simulink model "test_mdl1"  (R2023a)
settings: Solver=VariableStepAuto  StartTime=0.0  StopTime=10.0  RelTol=1e-3
(part 2 of 8)

== system test_mdl1/VehicleCAN/ABS_ESC/ABS_Rapid_Data_Response_2 ==
  UUDTABSResponse2 : Constant  Value=0
  bus_creator : BusCreator  Inputs=1
  out_port : Outport
  wires:
  bus_creator/1 -> out_port/1  "test_mdl1"
  UUDTABSResponse2/1 -> bus_creator/1  "UUDTABSResponse2"

== system test_mdl1/VehicleCAN/ABS_ESC/ActiveFronSteering_Req ==
  SteWhlBrkAnRq_No_Cnt : Constant  Value=0
  SteWhlBrkAnRq_No_Cs : Constant  Value=0
  SteWhlBrkOffst_An_Rq : Constant  Value=0
  bus_creator : BusCreator  Inputs=3
  out_port : Outport
  wires:
  bus_creator/1 -> out_port/1  "test_mdl1"
  SteWhlBrkAnRq_No_Cnt/1 -> bus_creator/1  "SteWhlBrkAnRq_No_Cnt"
  SteWhlBrkAnRq_No_Cs/1 -> bus_creator/2  "SteWhlBrkAnRq_No_Cs"
  SteWhlBrkOffst_An_Rq/1 -> bus_creator/3  "SteWhlBrkOffst_An_Rq"

== system test_mdl1/VehicleCAN/ABS_ESC/BrakeSnData_3 ==
  VehLatComp_A_Actl : Constant  Value=0
  VehLongComp_A_Actl : Constant  Value=0
  VehOverGnd_V_Est : Constant  Value=0
  VehTrvlDir_D_Stat : Constant  Value=0
  VehYawComp_W_Actl : Constant  Value=0
  bus_creator : BusCreator  Inputs=5
  out_port : Outport
  wires:
  bus_creator/1 -> out_port/1  "test_mdl1"
  VehLatComp_A_Actl/1 -> bus_creator/1  "VehLatComp_A_Actl"
  VehLongComp_A_Actl/1 -> bus_creator/2  "VehLongComp_A_Actl"
  VehOverGnd_V_Est/1 -> bus_creator/3  "VehOverGnd_V_Est"
  VehTrvlDir_D_Stat/1 -> bus_creator/4  "VehTrvlDir_D_Stat"
  VehYawComp_W_Actl/1 -> bus_creator/5  "VehYawComp_W_Actl"

== system test_mdl1/VehicleCAN/ABS_ESC/BrakeSnData_4 ==
  BrkTotTqRqArb_No_Cnt : Constant  Value=0
  BrkTotTqRqArb_No_Cs : Constant  Value=0
  BrkTot_Tq_Actl : Constant  Value=0
  BrkTot_Tq_RqArb : Constant  Value=0
  HsaStat_D_Actl : Constant  Value=0
  VehRolComp_W_Actl : Constant  Value=0
  VehVertComp_A_Actl : Constant  Value=0
  bus_creator : BusCreator  Inputs=7
  out_port : Outport
  wires:
  bus_creator/1 -> out_port/1  "test_mdl1"
  BrkTotTqRqArb_No_Cnt/1 -> bus_creator/1  "BrkTotTqRqArb_No_Cnt"
  BrkTotTqRqArb_No_Cs/1 -> bus_creator/2  "BrkTotTqRqArb_No_Cs"
  BrkTot_Tq_Actl/1 -> bus_creator/3  "BrkTot_Tq_Actl"
  BrkTot_Tq_RqArb/1 -> bus_creator/4  "BrkTot_Tq_RqArb"
  HsaStat_D_Actl/1 -> bus_creator/5  "HsaStat_D_Actl"
  VehRolComp_W_Actl/1 -> bus_creator/6  "VehRolComp_W_Actl"
  VehVertComp_A_Actl/1 -> bus_creator/7  "VehVertComp_A_Actl"

== system test_mdl1/VehicleCAN/ABS_ESC/BrakeSnData_5 ==
  AwdLck_Tq_RqMn : Constant  Value=0
  AwdLck_Tq_RqMx : Constant  Value=0
  BrkCtrFnd_B_Stat : Constant  Value=0
  DrvSte_D_Stat : Constant  Value=0
  DrvSte_Tq_Rq : Constant  Value=0
  EmgcyBrkLamp_D_Rq : Constant  Value=0
  StopLamp_B_RqBrk : Constant  Value=0
  bus_creator : BusCreator  Inputs=7
  out_port : Outport
  wires:
  bus_creator/1 -> out_port/1  "test_mdl1"
  AwdLck_Tq_RqMn/1 -> bus_creator/1  "AwdLck_Tq_RqMn"
  AwdLck_Tq_RqMx/1 -> bus_creator/2  "AwdLck_Tq_RqMx"
  BrkCtrFnd_B_Stat/1 -> bus_creator/3  "BrkCtrFnd_B_Stat"
  DrvSte_D_Stat/1 -> bus_creator/4  "DrvSte_D_Stat"
  DrvSte_Tq_Rq/1 -> bus_creator/5  "DrvSte_Tq_Rq"
  EmgcyBrkLamp_D_Rq/1 -> bus_creator/6  "EmgcyBrkLamp_D_Rq"
  StopLamp_B_RqBrk/1 -> bus_creator/7  "StopLamp_B_RqBrk"

== system test_mdl1/VehicleCAN/ABS_ESC/BrakeSnData_6 ==
  StePinOffst_An_Est : Constant  Value=0
  StePinOffst_D_Stat : Constant  Value=0
  StePinOffst_No_Cnt : Constant  Value=0
  StePinOffst_No_Cs : Constant  Value=0
  bus_creator : BusCreator  Inputs=4
  out_port : Outport
  wires:
  bus_creator/1 -> out_port/1  "test_mdl1"
  StePinOffst_An_Est/1 -> bus_creator/1  "StePinOffst_An_Est"
  StePinOffst_D_Stat/1 -> bus_creator/2  "StePinOffst_D_Stat"
  StePinOffst_No_Cnt/1 -> bus_creator/3  "StePinOffst_No_Cnt"
  StePinOffst_No_Cs/1 -> bus_creator/4  "StePinOffst_No_Cs"

== system test_mdl1/VehicleCAN/ABS_ESC/BrakeSysFeatures ==
  BrkFluidLvl_D_Stat : Constant  Value=0
  LsmcBrkDecel_D_Stat : Constant  Value=0
  VehStab_D_Stat : Constant  Value=0
  VehVActlBrk_D_Qf : Constant  Value=0
  VehVActlBrk_No_Cnt : Constant  Value=0
  VehVActlBrk_No_Cs : Constant  Value=0
  VehYawLin_W_Rq : Constant  Value=0
  VehYawNonLin_W_Rq : Constant  Value=0
  Veh_V_ActlBrk : Constant  Value=0
  bus_creator : BusCreator  Inputs=9
  out_port : Outport
  wires:
  bus_creator/1 -> out_port/1  "test_mdl1"
  BrkFluidLvl_D_Stat/1 -> bus_creator/1  "BrkFluidLvl_D_Stat"
  LsmcBrkDecel_D_Stat/1 -> bus_creator/2  "LsmcBrkDecel_D_Stat"
  VehStab_D_Stat/1 -> bus_creator/3  "VehStab_D_Stat"
  VehVActlBrk_D_Qf/1 -> bus_creator/4  "VehVActlBrk_D_Qf"
  VehVActlBrk_No_Cnt/1 -> bus_creator/5  "VehVActlBrk_No_Cnt"
  VehVActlBrk_No_Cs/1 -> bus_creator/6  "VehVActlBrk_No_Cs"
  VehYawLin_W_Rq/1 -> bus_creator/7  "VehYawLin_W_Rq"
  VehYawNonLin_W_Rq/1 -> bus_creator/8  "VehYawNonLin_W_Rq"
  Veh_V_ActlBrk/1 -> bus_creator/9  "Veh_V_ActlBrk"

== system test_mdl1/VehicleCAN/ABS_ESC/BrakeSysFeatures_2 ==
  Abs_B_Falt : Constant  Value=0
  BpedMove_D_Actl : Constant  Value=0
  BpedMove_No_Cnt : Constant  Value=0
  BrkBstrVac_B_Rq : Constant  Value=0
  BrkLamp_B_Rq : Constant  Value=0
  ChimeBrk_B_Rq : Constant  Value=0
  DrvAntiLckLamp_D_Rq : Constant  Value=0
  DrvHdcLampInfo_D_Rq : Constant  Value=0
  DrvHdcMsg_D_Rq : Constant  Value=0
  DrvHdcWarnInfo_D_Rq : Constant  Value=0
  DrvSlipCtlLamp_D_Rq : Constant  Value=0
  DrvSlipCtlMde_D_Ind : Constant  Value=0
  HILL_DESC_MC : Constant  Value=0
  HdcMde_D_Actl : Constant  Value=0
  HsaMde_D_Mem : Constant  Value=0
  RearDiffElckrOpen_B_Rq : Constant  Value=0
  RearDiffLck_Tq2_RqMx : Constant  Value=0
  StabCtlBrk_B_Avail : Constant  Value=0
  TCMode : Constant  Value=0
  TRLR_SWAY_CONFIG_STAT : Constant  Value=0
  TRLR_SWAY_EVNT_IN_PROG : Constant  Value=0
  bus_creator : BusCreator  Inputs=21
  out_port : Outport
  wires:
  bus_creator/1 -> out_port/1  "test_mdl1"
  Abs_B_Falt/1 -> bus_creator/1  "Abs_B_Falt"
  BpedMove_D_Actl/1 -> bus_creator/2  "BpedMove_D_Actl"
  BpedMove_No_Cnt/1 -> bus_creator/3  "BpedMove_No_Cnt"
  BrkBstrVac_B_Rq/1 -> bus_creator/4  "BrkBstrVac_B_Rq"
  BrkLamp_B_Rq/1 -> bus_creator/5  "BrkLamp_B_Rq"
  ChimeBrk_B_Rq/1 -> bus_creator/6  "ChimeBrk_B_Rq"
  DrvAntiLckLamp_D_Rq/1 -> bus_creator/7  "DrvAntiLckLamp_D_Rq"
  DrvHdcLampInfo_D_Rq/1 -> bus_creator/8  "DrvHdcLampInfo_D_Rq"
  DrvHdcMsg_D_Rq/1 -> bus_creator/9  "DrvHdcMsg_D_Rq"
  DrvHdcWarnInfo_D_Rq/1 -> bus_creator/10  "DrvHdcWarnInfo_D_Rq"
  DrvSlipCtlLamp_D_Rq/1 -> bus_creator/11  "DrvSlipCtlLamp_D_Rq"
  DrvSlipCtlMde_D_Ind/1 -> bus_creator/12  "DrvSlipCtlMde_D_Ind"
  HILL_DESC_MC/1 -> bus_creator/13  "HILL_DESC_MC"
  HdcMde_D_Actl/1 -> bus_creator/14  "HdcMde_D_Actl"
  HsaMde_D_Mem/1 -> bus_creator/15  "HsaMde_D_Mem"
  RearDiffElckrOpen_B_Rq/1 -> bus_creator/16  "RearDiffElckrOpen_B_Rq"
  RearDiffLck_Tq2_RqMx/1 -> bus_creator/17  "RearDiffLck_Tq2_RqMx"
  StabCtlBrk_B_Avail/1 -> bus_creator/18  "StabCtlBrk_B_Avail"
  TCMode/1 -> bus_creator/19  "TCMode"
  TRLR_SWAY_CONFIG_STAT/1 -> bus_creator/20  "TRLR_SWAY_CONFIG_STAT"
  TRLR_SWAY_EVNT_IN_PROG/1 -> bus_creator/21  "TRLR_SWAY_EVNT_IN_PROG"

== system test_mdl1/VehicleCAN/ABS_ESC/BrakeSysFeatures_3 ==
  AirDamUp_B_RqBrk : Constant  Value=0
  ApaBrk_D_Stat : Constant  Value=0
  AutoHoldMde_D_Ind : Constant  Value=0
  AutoHoldMsgTxt_D_Rq : Constant  Value=0
  AutoHoldSwMde_B_Ind : Constant  Value=0
  BrkBstrVac_D_Stat : Constant  Value=0
  CtaBrk_D_Stat : Constant  Value=0
  DrvSlipCtlMdeMsg_D_Rq : Constant  Value=0
  DrvSlipCtlOffLamp_D_Rq : Constant  Value=0
  RbaBrk_D_Stat : Constant  Value=0
  SelDrvMdeAwd_D_Rq : Constant  Value=0
  SelDrvMdeChassis2_D_Rq : Constant  Value=0
  SelDrvMdeChassis_D_Rq : Constant  Value=0
  TrailCtlMsgTxt_D_Rq : Constant  Value=0
  TrailCtl_D_Stat : Constant  Value=0
  bus_creator : BusCreator  Inputs=15
  out_port : Outport
  wires:
  bus_creator/1 -> out_port/1  "test_mdl1"
  AirDamUp_B_RqBrk/1 -> bus_creator/1  "AirDamUp_B_RqBrk"
  ApaBrk_D_Stat/1 -> bus_creator/2  "ApaBrk_D_Stat"
  AutoHoldMde_D_Ind/1 -> bus_creator/3  "AutoHoldMde_D_Ind"
  AutoHoldMsgTxt_D_Rq/1 -> bus_creator/4  "AutoHoldMsgTxt_D_Rq"
  AutoHoldSwMde_B_Ind/1 -> bus_creator/5  "AutoHoldSwMde_B_Ind"
  BrkBstrVac_D_Stat/1 -> bus_creator/6  "BrkBstrVac_D_Stat"
  CtaBrk_D_Stat/1 -> bus_creator/7  "CtaBrk_D_Stat"
  DrvSlipCtlMdeMsg_D_Rq/1 -> bus_creator/8  "DrvSlipCtlMdeMsg_D_Rq"
  DrvSlipCtlOffLamp_D_Rq/1 -> bus_creator/9  "DrvSlipCtlOffLamp_D_Rq"
  RbaBrk_D_Stat/1 -> bus_creator/10  "RbaBrk_D_Stat"
  SelDrvMdeAwd_D_Rq/1 -> bus_creator/11  "SelDrvMdeAwd_D_Rq"
  SelDrvMdeChassis2_D_Rq/1 -> bus_creator/12  "SelDrvMdeChassis2_D_Rq"
  SelDrvMdeChassis_D_Rq/1 -> bus_creator/13  "SelDrvMdeChassis_D_Rq"
  TrailCtlMsgTxt_D_Rq/1 -> bus_creator/14  "TrailCtlMsgTxt_D_Rq"
  TrailCtl_D_Stat/1 -> bus_creator/15  "TrailCtl_D_Stat"

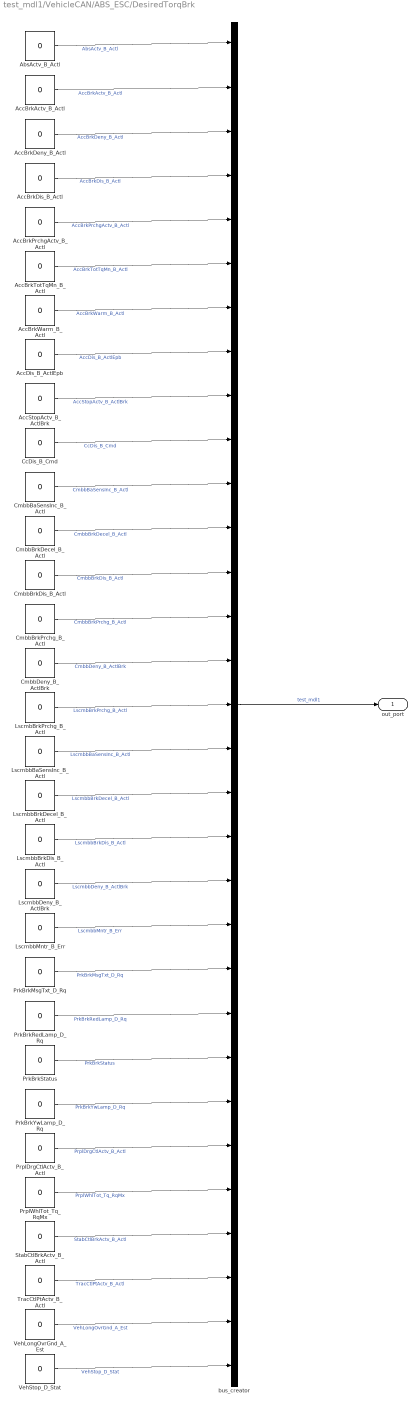
== system test_mdl1/VehicleCAN/ABS_ESC/DesiredTorqBrk ==
  AbsActv_B_Actl : Constant  Value=0
  AccBrkActv_B_Actl : Constant  Value=0
  AccBrkDeny_B_Actl : Constant  Value=0
  AccBrkDis_B_Actl : Constant  Value=0
  AccBrkPrchgActv_B_Actl : Constant  Value=0
  AccBrkTotTqMn_B_Actl : Constant  Value=0
  AccBrkWarm_B_Actl : Constant  Value=0
  AccDis_B_ActlEpb : Constant  Value=0
  AccStopActv_B_ActlBrk : Constant  Value=0
  CcDis_B_Cmd : Constant  Value=0
  CmbbBaSensInc_B_Actl : Constant  Value=0
  CmbbBrkDecel_B_Actl : Constant  Value=0
  CmbbBrkDis_B_Actl : Constant  Value=0
  CmbbBrkPrchg_B_Actl : Constant  Value=0
  CmbbDeny_B_ActlBrk : Constant  Value=0
  LscmbBrkPrchg_B_Actl : Constant  Value=0
  LscmbbBaSensInc_B_Actl : Constant  Value=0
  LscmbbBrkDecel_B_Actl : Constant  Value=0
  LscmbbBrkDis_B_Actl : Constant  Value=0
  LscmbbDeny_B_ActlBrk : Constant  Value=0
  LscmbbMntr_B_Err : Constant  Value=0
  PrkBrkMsgTxt_D_Rq : Constant  Value=0
  PrkBrkRedLamp_D_Rq : Constant  Value=0
  PrkBrkStatus : Constant  Value=0
  PrkBrkYwLamp_D_Rq : Constant  Value=0
  PrplDrgCtlActv_B_Actl : Constant  Value=0
  PrplWhlTot_Tq_RqMx : Constant  Value=0
  StabCtlBrkActv_B_Actl : Constant  Value=0
  TracCtlPtActv_B_Actl : Constant  Value=0
  VehLongOvrGnd_A_Est : Constant  Value=0
  VehStop_D_Stat : Constant  Value=0
  bus_creator : BusCreator  Inputs=31
  out_port : Outport
  wires:
  bus_creator/1 -> out_port/1  "test_mdl1"
  AbsActv_B_Actl/1 -> bus_creator/1  "AbsActv_B_Actl"
  AccBrkActv_B_Actl/1 -> bus_creator/2  "AccBrkActv_B_Actl"
  AccBrkDeny_B_Actl/1 -> bus_creator/3  "AccBrkDeny_B_Actl"
  AccBrkDis_B_Actl/1 -> bus_creator/4  "AccBrkDis_B_Actl"
  AccBrkPrchgActv_B_Actl/1 -> bus_creator/5  "AccBrkPrchgActv_B_Actl"
  AccBrkTotTqMn_B_Actl/1 -> bus_creator/6  "AccBrkTotTqMn_B_Actl"
  AccBrkWarm_B_Actl/1 -> bus_creator/7  "AccBrkWarm_B_Actl"
  AccDis_B_ActlEpb/1 -> bus_creator/8  "AccDis_B_ActlEpb"
  AccStopActv_B_ActlBrk/1 -> bus_creator/9  "AccStopActv_B_ActlBrk"
  CcDis_B_Cmd/1 -> bus_creator/10  "CcDis_B_Cmd"
  CmbbBaSensInc_B_Actl/1 -> bus_creator/11  "CmbbBaSensInc_B_Actl"
  CmbbBrkDecel_B_Actl/1 -> bus_creator/12  "CmbbBrkDecel_B_Actl"
  CmbbBrkDis_B_Actl/1 -> bus_creator/13  "CmbbBrkDis_B_Actl"
  CmbbBrkPrchg_B_Actl/1 -> bus_creator/14  "CmbbBrkPrchg_B_Actl"
  CmbbDeny_B_ActlBrk/1 -> bus_creator/15  "CmbbDeny_B_ActlBrk"
  LscmbBrkPrchg_B_Actl/1 -> bus_creator/16  "LscmbBrkPrchg_B_Actl"
  LscmbbBaSensInc_B_Actl/1 -> bus_creator/17  "LscmbbBaSensInc_B_Actl"
  LscmbbBrkDecel_B_Actl/1 -> bus_creator/18  "LscmbbBrkDecel_B_Actl"
  LscmbbBrkDis_B_Actl/1 -> bus_creator/19  "LscmbbBrkDis_B_Actl"
  LscmbbDeny_B_ActlBrk/1 -> bus_creator/20  "LscmbbDeny_B_ActlBrk"
  LscmbbMntr_B_Err/1 -> bus_creator/21  "LscmbbMntr_B_Err"
  PrkBrkMsgTxt_D_Rq/1 -> bus_creator/22  "PrkBrkMsgTxt_D_Rq"
  PrkBrkRedLamp_D_Rq/1 -> bus_creator/23  "PrkBrkRedLamp_D_Rq"
  PrkBrkStatus/1 -> bus_creator/24  "PrkBrkStatus"
  PrkBrkYwLamp_D_Rq/1 -> bus_creator/25  "PrkBrkYwLamp_D_Rq"
  PrplDrgCtlActv_B_Actl/1 -> bus_creator/26  "PrplDrgCtlActv_B_Actl"
  PrplWhlTot_Tq_RqMx/1 -> bus_creator/27  "PrplWhlTot_Tq_RqMx"
  StabCtlBrkActv_B_Actl/1 -> bus_creator/28  "StabCtlBrkActv_B_Actl"
  TracCtlPtActv_B_Actl/1 -> bus_creator/29  "TracCtlPtActv_B_Actl"
  VehLongOvrGnd_A_Est/1 -> bus_creator/30  "VehLongOvrGnd_A_Est"
  VehStop_D_Stat/1 -> bus_creator/31  "VehStop_D_Stat"

== system test_mdl1/VehicleCAN/ABS_ESC/DesiredTorqBrk_2 ==
  PrplWhlTot_Tq_RqMn : Constant  Value=0
  PrplWhlTqRqMn_No_Cnt : Constant  Value=0
  PrplWhlTqRqMn_No_Cs : Constant  Value=0
  RgenBrkDynoMde_B_Actl : Constant  Value=0
  RgenTqFalt_B_Actl : Constant  Value=0
  bus_creator : BusCreator  Inputs=5
  out_port : Outport
  wires:
  bus_creator/1 -> out_port/1  "test_mdl1"
  PrplWhlTot_Tq_RqMn/1 -> bus_creator/1  "PrplWhlTot_Tq_RqMn"
  PrplWhlTqRqMn_No_Cnt/1 -> bus_creator/2  "PrplWhlTqRqMn_No_Cnt"
  PrplWhlTqRqMn_No_Cs/1 -> bus_creator/3  "PrplWhlTqRqMn_No_Cs"
  RgenBrkDynoMde_B_Actl/1 -> bus_creator/4  "RgenBrkDynoMde_B_Actl"
  RgenTqFalt_B_Actl/1 -> bus_creator/5  "RgenTqFalt_B_Actl"

== system test_mdl1/VehicleCAN/ABS_ESC/Global_PATS_SubTarget ==
  bus_creator : BusCreator  Inputs=2
  immoSubTarget1Cmd_T1 : Constant  Value=0
  immoSubTarget1Data_T1 : Constant  Value=0
  out_port : Outport
  wires:
  bus_creator/1 -> out_port/1  "test_mdl1"
  immoSubTarget1Cmd_T1/1 -> bus_creator/1  "immoSubTarget1Cmd_T1"
  immoSubTarget1Data_T1/1 -> bus_creator/2  "immoSubTarget1Data_T1"

== system test_mdl1/VehicleCAN/ABS_ESC/OTAPhysABStoGWM_ECG ==
  OTAPhysABStoGWM_ECG : Constant  Value=0
  bus_creator : BusCreator  Inputs=1
  out_port : Outport
  wires:
  bus_creator/1 -> out_port/1  "test_mdl1"
  OTAPhysABStoGWM_ECG/1 -> bus_creator/1  "OTAPhysABStoGWM_ECG"

== system test_mdl1/VehicleCAN/ABS_ESC/PARSEDPhysABStoGWM_ECG ==
  PARSEDPhysABStoGWM_ECG : Constant  Value=0
  bus_creator : BusCreator  Inputs=1
  out_port : Outport
  wires:
  bus_creator/1 -> out_port/1  "test_mdl1"
  PARSEDPhysABStoGWM_ECG/1 -> bus_creator/1  "PARSEDPhysABStoGWM_ECG"

== system test_mdl1/VehicleCAN/ABS_ESC/PARSEDPushABStoGWM_ECG ==
  PARSEDPhysABS2toGWM_ECG : Constant  Value=0
  bus_creator : BusCreator  Inputs=1
  out_port : Outport
  wires:
  bus_creator/1 -> out_port/1  "test_mdl1"
  PARSEDPhysABS2toGWM_ECG/1 -> bus_creator/1  "PARSEDPhysABS2toGWM_ECG"

== system test_mdl1/VehicleCAN/ABS_ESC/SelectDriveModeData ==
  ActvDrvMde_D2_Stat : Constant  Value=0
  AutoEpbButtnOn_B_Stat : Constant  Value=0
  AutoEpbDsply_D_Stat : Constant  Value=0
  AutoEpbMsgTxt_D_Rq : Constant  Value=0
  AwdMde_D_RqBrk : Constant  Value=0
  SelDrvMdeMsgTxt_D_Rq : Constant  Value=0
  SelDrvMdePos01_B_Avail : Constant  Value=0
  SelDrvMdePos02_B_Avail : Constant  Value=0
  SelDrvMdePos03_B_Avail : Constant  Value=0
  SelDrvMdePos04_B_Avail : Constant  Value=0
  SelDrvMdePos05_B_Avail : Constant  Value=0
  SelDrvMdePos06_B_Avail : Constant  Value=0
  SelDrvMdePos07_B_Avail : Constant  Value=0
  SelDrvMdePos08_B_Avail : Constant  Value=0
  SelDrvMdePos09_B_Avail : Constant  Value=0
  SelDrvMdePos10_B_Avail : Constant  Value=0
  SelDrvMdePos11_B_Avail : Constant  Value=0
  SelDrvMdePos12_B_Avail : Constant  Value=0
  SelDrvMdePt_D_Rq : Constant  Value=0
  SelDrvMde_D2_Rq : Constant  Value=0
  SelDrvMde_D_Stat : Constant  Value=0
  bus_creator : BusCreator  Inputs=21
  out_port : Outport
  wires:
  bus_creator/1 -> out_port/1  "test_mdl1"
  ActvDrvMde_D2_Stat/1 -> bus_creator/1  "ActvDrvMde_D2_Stat"
  AutoEpbButtnOn_B_Stat/1 -> bus_creator/2  "AutoEpbButtnOn_B_Stat"
  AutoEpbDsply_D_Stat/1 -> bus_creator/3  "AutoEpbDsply_D_Stat"
  AutoEpbMsgTxt_D_Rq/1 -> bus_creator/4  "AutoEpbMsgTxt_D_Rq"
  AwdMde_D_RqBrk/1 -> bus_creator/5  "AwdMde_D_RqBrk"
  SelDrvMdeMsgTxt_D_Rq/1 -> bus_creator/6  "SelDrvMdeMsgTxt_D_Rq"
  SelDrvMdePos01_B_Avail/1 -> bus_creator/7  "SelDrvMdePos01_B_Avail"
  SelDrvMdePos02_B_Avail/1 -> bus_creator/8  "SelDrvMdePos02_B_Avail"
  SelDrvMdePos03_B_Avail/1 -> bus_creator/9  "SelDrvMdePos03_B_Avail"
  SelDrvMdePos04_B_Avail/1 -> bus_creator/10  "SelDrvMdePos04_B_Avail"
  SelDrvMdePos05_B_Avail/1 -> bus_creator/11  "SelDrvMdePos05_B_Avail"
  SelDrvMdePos06_B_Avail/1 -> bus_creator/12  "SelDrvMdePos06_B_Avail"
  SelDrvMdePos07_B_Avail/1 -> bus_creator/13  "SelDrvMdePos07_B_Avail"
  SelDrvMdePos08_B_Avail/1 -> bus_creator/14  "SelDrvMdePos08_B_Avail"
  SelDrvMdePos09_B_Avail/1 -> bus_creator/15  "SelDrvMdePos09_B_Avail"
  SelDrvMdePos10_B_Avail/1 -> bus_creator/16  "SelDrvMdePos10_B_Avail"
  SelDrvMdePos11_B_Avail/1 -> bus_creator/17  "SelDrvMdePos11_B_Avail"
  SelDrvMdePos12_B_Avail/1 -> bus_creator/18  "SelDrvMdePos12_B_Avail"
  SelDrvMdePt_D_Rq/1 -> bus_creator/19  "SelDrvMdePt_D_Rq"
  SelDrvMde_D2_Rq/1 -> bus_creator/20  "SelDrvMde_D2_Rq"
  SelDrvMde_D_Stat/1 -> bus_creator/21  "SelDrvMde_D_Stat"

== system test_mdl1/VehicleCAN/ABS_ESC/SelectDriveModeData2 ==
  SelDrvMdePos01_D_Stat : Constant  Value=0
  SelDrvMdePos02_D_Stat : Constant  Value=0
  SelDrvMdePos03_D_Stat : Constant  Value=0
  SelDrvMdePos04_D_Stat : Constant  Value=0
  SelDrvMdePos05_D_Stat : Constant  Value=0
  SelDrvMdePos06_D_Stat : Constant  Value=0
  SelDrvMdePos07_D_Stat : Constant  Value=0
  SelDrvMdePos08_D_Stat : Constant  Value=0
  SelDrvMdePos09_D_Stat : Constant  Value=0
  SelDrvMdePos10_D_Stat : Constant  Value=0
  SelDrvMdePos11_D_Stat : Constant  Value=0
  SelDrvMdePos12_D_Stat : Constant  Value=0
  bus_creator : BusCreator  Inputs=12
  out_port : Outport
  wires:
  bus_creator/1 -> out_port/1  "test_mdl1"
  SelDrvMdePos01_D_Stat/1 -> bus_creator/1  "SelDrvMdePos01_D_Stat"
  SelDrvMdePos02_D_Stat/1 -> bus_creator/2  "SelDrvMdePos02_D_Stat"
  SelDrvMdePos03_D_Stat/1 -> bus_creator/3  "SelDrvMdePos03_D_Stat"
  SelDrvMdePos04_D_Stat/1 -> bus_creator/4  "SelDrvMdePos04_D_Stat"
  SelDrvMdePos05_D_Stat/1 -> bus_creator/5  "SelDrvMdePos05_D_Stat"
  SelDrvMdePos06_D_Stat/1 -> bus_creator/6  "SelDrvMdePos06_D_Stat"
  SelDrvMdePos07_D_Stat/1 -> bus_creator/7  "SelDrvMdePos07_D_Stat"
  SelDrvMdePos08_D_Stat/1 -> bus_creator/8  "SelDrvMdePos08_D_Stat"
  SelDrvMdePos09_D_Stat/1 -> bus_creator/9  "SelDrvMdePos09_D_Stat"
  SelDrvMdePos10_D_Stat/1 -> bus_creator/10  "SelDrvMdePos10_D_Stat"
  SelDrvMdePos11_D_Stat/1 -> bus_creator/11  "SelDrvMdePos11_D_Stat"
  SelDrvMdePos12_D_Stat/1 -> bus_creator/12  "SelDrvMdePos12_D_Stat"

== system test_mdl1/VehicleCAN/ABS_ESC/TesterPhysicalResABS ==
  TesterPhysicalResABS : Constant  Value=0
  bus_creator : BusCreator  Inputs=1
  out_port : Outport
  wires:
  bus_creator/1 -> out_port/1  "test_mdl1"
  TesterPhysicalResABS/1 -> bus_creator/1  "TesterPhysicalResABS"

== system test_mdl1/VehicleCAN/ABS_ESC/TrailerBrakeData ==
  TrlrBrk_Pc_Rq : Constant  Value=0
  VehPtch_An_Dsply : Constant  Value=0
  VehRol_An_Dsply : Constant  Value=0
  bus_creator : BusCreator  Inputs=3
  out_port : Outport
  wires:
  bus_creator/1 -> out_port/1  "test_mdl1"
  TrlrBrk_Pc_Rq/1 -> bus_creator/1  "TrlrBrk_Pc_Rq"
  VehPtch_An_Dsply/1 -> bus_creator/2  "VehPtch_An_Dsply"
  VehRol_An_Dsply/1 -> bus_creator/3  "VehRol_An_Dsply"

== system test_mdl1/VehicleCAN/ABS_ESC/WheelData ==
  BrkObdData_No_Actl : Constant  Value=0
  BrkObdIndex_No_Actl : Constant  Value=0
  WhlDirFl_D_Actl : Constant  Value=0
  WhlDirFr_D_Actl : Constant  Value=0
  WhlDirRl_D_Actl : Constant  Value=0
  WhlDirRr_D_Actl : Constant  Value=0
  WhlRotatFl_No_Cnt : Constant  Value=0
  WhlRotatFr_No_Cnt : Constant  Value=0
  WhlRotatRl_No_Cnt : Constant  Value=0
  WhlRotatRr_No_Cnt : Constant  Value=0
  bus_creator : BusCreator  Inputs=10
  out_port : Outport
  wires:
  bus_creator/1 -> out_port/1  "test_mdl1"
  BrkObdData_No_Actl/1 -> bus_creator/1  "BrkObdData_No_Actl"
  BrkObdIndex_No_Actl/1 -> bus_creator/2  "BrkObdIndex_No_Actl"
  WhlDirFl_D_Actl/1 -> bus_creator/3  "WhlDirFl_D_Actl"
  WhlDirFr_D_Actl/1 -> bus_creator/4  "WhlDirFr_D_Actl"
  WhlDirRl_D_Actl/1 -> bus_creator/5  "WhlDirRl_D_Actl"
  WhlDirRr_D_Actl/1 -> bus_creator/6  "WhlDirRr_D_Actl"
  WhlRotatFl_No_Cnt/1 -> bus_creator/7  "WhlRotatFl_No_Cnt"
  WhlRotatFr_No_Cnt/1 -> bus_creator/8  "WhlRotatFr_No_Cnt"
  WhlRotatRl_No_Cnt/1 -> bus_creator/9  "WhlRotatRl_No_Cnt"
  WhlRotatRr_No_Cnt/1 -> bus_creator/10  "WhlRotatRr_No_Cnt"

== system test_mdl1/VehicleCAN/ABS_ESC/WheelSpeed ==
  WhlFl_W_Meas : Constant  Value=0
  WhlFr_W_Meas : Constant  Value=0
  WhlRl_W_Meas : Constant  Value=0
  WhlRr_W_Meas : Constant  Value=0
  bus_creator : BusCreator  Inputs=4
  out_port : Outport
  wires:
  bus_creator/1 -> out_port/1  "test_mdl1"
  WhlFl_W_Meas/1 -> bus_creator/1  "WhlFl_W_Meas"
  WhlFr_W_Meas/1 -> bus_creator/2  "WhlFr_W_Meas"
  WhlRl_W_Meas/1 -> bus_creator/3  "WhlRl_W_Meas"
  WhlRr_W_Meas/1 -> bus_creator/4  "WhlRr_W_Meas"

== system test_mdl1/VehicleCAN/CMR_DSMC/CMR_DSMC_AutoSar_NetwrkMgt ==
  CMR_DSMC_AutoSarNMControl : Constant  Value=0
  CMR_DSMC_AutoSarNMNodeId : Constant  Value=0
  CMR_DSMC_AutoSarNMReserve2 : Constant  Value=0
  CMR_DSMC_AutoSarNMReserve3 : Constant  Value=0
  CMR_DSMC_AutoSarNMReserve4 : Constant  Value=0
  CMR_DSMC_AutoSarNMReserved : Constant  Value=0
  CMR_DSMC_GWNMProxY : Constant  Value=0
  CMR_DSMC_GWOnBoardTester : Constant  Value=0
  bus_creator : BusCreator  Inputs=8
  out_port : Outport
  wires:
  bus_creator/1 -> out_port/1  "test_mdl1"
  CMR_DSMC_AutoSarNMControl/1 -> bus_creator/1  "CMR_DSMC_AutoSarNMControl"
  CMR_DSMC_AutoSarNMNodeId/1 -> bus_creator/2  "CMR_DSMC_AutoSarNMNodeId"
  CMR_DSMC_AutoSarNMReserve2/1 -> bus_creator/3  "CMR_DSMC_AutoSarNMReserve2"
  CMR_DSMC_AutoSarNMReserve3/1 -> bus_creator/4  "CMR_DSMC_AutoSarNMReserve3"
  CMR_DSMC_AutoSarNMReserve4/1 -> bus_creator/5  "CMR_DSMC_AutoSarNMReserve4"
  CMR_DSMC_AutoSarNMReserved/1 -> bus_creator/6  "CMR_DSMC_AutoSarNMReserved"
  CMR_DSMC_GWNMProxY/1 -> bus_creator/7  "CMR_DSMC_GWNMProxY"
  CMR_DSMC_GWOnBoardTester/1 -> bus_creator/8  "CMR_DSMC_GWOnBoardTester"

== system test_mdl1/VehicleCAN/CMR_DSMC/DrvStatMonData ==
  DrvAlertSt_D_Stat : Constant  Value=0
  DrvAttentZone_D_Stat : Constant  Value=0
  DrvCamDrvIR_D_Stat : Constant  Value=0
  DrvCamPassIR_D_Stat : Constant  Value=0
  DrvCamera_D_Stat : Constant  Value=0
  DrvEngLvlConfid_D_Stat : Constant  Value=0
  DrvEngageLevel_D_Stat : Constant  Value=0
  DrvEngageLevel_No_Cnt : Constant  Value=0
  DrvEngageLevel_No_Cs : Constant  Value=0
  DrvImpLvlConfid_D_Stat : Constant  Value=0
  DrvImpairLvl_D_Stat : Constant  Value=0
  bus_creator : BusCreator  Inputs=11
  out_port : Outport
  wires:
  bus_creator/1 -> out_port/1  "test_mdl1"
  DrvAlertSt_D_Stat/1 -> bus_creator/1  "DrvAlertSt_D_Stat"
  DrvAttentZone_D_Stat/1 -> bus_creator/2  "DrvAttentZone_D_Stat"
  DrvCamDrvIR_D_Stat/1 -> bus_creator/3  "DrvCamDrvIR_D_Stat"
  DrvCamPassIR_D_Stat/1 -> bus_creator/4  "DrvCamPassIR_D_Stat"
  DrvCamera_D_Stat/1 -> bus_creator/5  "DrvCamera_D_Stat"
  DrvEngLvlConfid_D_Stat/1 -> bus_creator/6  "DrvEngLvlConfid_D_Stat"
  DrvEngageLevel_D_Stat/1 -> bus_creator/7  "DrvEngageLevel_D_Stat"
  DrvEngageLevel_No_Cnt/1 -> bus_creator/8  "DrvEngageLevel_No_Cnt"
  DrvEngageLevel_No_Cs/1 -> bus_creator/9  "DrvEngageLevel_No_Cs"
  DrvImpLvlConfid_D_Stat/1 -> bus_creator/10  "DrvImpLvlConfid_D_Stat"
  DrvImpairLvl_D_Stat/1 -> bus_creator/11  "DrvImpairLvl_D_Stat"

== system test_mdl1/VehicleCAN/CMR_DSMC/TesterPhysicalResCMR_DSMC ==
  TesterPhysicalResCMR_DSMC : Constant  Value=0
  bus_creator : BusCreator  Inputs=1
  out_port : Outport
  wires:
  bus_creator/1 -> out_port/1  "test_mdl1"
  TesterPhysicalResCMR_DSMC/1 -> bus_creator/1  "TesterPhysicalResCMR_DSMC"

== system test_mdl1/VehicleCAN/ECM_Diesel/CGEA_Urea_Strategy ==
  DieslPrtcWarn_D_Rq : Constant  Value=0
  UreaLvlQlty_D_RqDsply : Constant  Value=0
  UreaLvlTxtWarn_D_Rq : Constant  Value=0
  UreaLvlTxt_D_RqDsply : Constant  Value=0
  UreaLvl_Pc_Actl : Constant  Value=0
  UreaQltyFlg_B_RqDsply : Constant  Value=0
  UreaQltySysWarn_D_Rq : Constant  Value=0
  UreaQltySys_D_RqDsply : Constant  Value=0
  VehUreaRnge2_L_DsplyMx : Constant  Value=0
  VehUreaWarn_V_DsplyMx : Constant  Value=0
  bus_creator : BusCreator  Inputs=10
  out_port : Outport
  wires:
  bus_creator/1 -> out_port/1  "test_mdl1"
  DieslPrtcWarn_D_Rq/1 -> bus_creator/1  "DieslPrtcWarn_D_Rq"
  UreaLvlQlty_D_RqDsply/1 -> bus_creator/2  "UreaLvlQlty_D_RqDsply"
  UreaLvlTxtWarn_D_Rq/1 -> bus_creator/3  "UreaLvlTxtWarn_D_Rq"
  UreaLvlTxt_D_RqDsply/1 -> bus_creator/4  "UreaLvlTxt_D_RqDsply"
  UreaLvl_Pc_Actl/1 -> bus_creator/5  "UreaLvl_Pc_Actl"
  UreaQltyFlg_B_RqDsply/1 -> bus_creator/6  "UreaQltyFlg_B_RqDsply"
  UreaQltySysWarn_D_Rq/1 -> bus_creator/7  "UreaQltySysWarn_D_Rq"
  UreaQltySys_D_RqDsply/1 -> bus_creator/8  "UreaQltySys_D_RqDsply"
  VehUreaRnge2_L_DsplyMx/1 -> bus_creator/9  "VehUreaRnge2_L_DsplyMx"
  VehUreaWarn_V_DsplyMx/1 -> bus_creator/10  "VehUreaWarn_V_DsplyMx"

== system test_mdl1/VehicleCAN/ECM_Diesel/EffDrvModeData ==
  EdmCmplnc_B_Dsply : Constant  Value=0
  EdmCmplnc_Pc_Dsply : Constant  Value=0
  EdmCurrent_Fe_Dsply : Constant  Value=0
  EdmLamp_D_Dsply : Constant  Value=0
  EdmMsgTxt_D_Rq : Constant  Value=0
  EdmPrev_Fe_Dsply : Constant  Value=0
  EdmSailMdeOn_B_Stat : Constant  Value=0
  EdmVeh_V_Dsply : Constant  Value=0
  bus_creator : BusCreator  Inputs=8
  out_port : Outport
  wires:
  bus_creator/1 -> out_port/1  "test_mdl1"
  EdmCmplnc_B_Dsply/1 -> bus_creator/1  "EdmCmplnc_B_Dsply"
  EdmCmplnc_Pc_Dsply/1 -> bus_creator/2  "EdmCmplnc_Pc_Dsply"
  EdmCurrent_Fe_Dsply/1 -> bus_creator/3  "EdmCurrent_Fe_Dsply"
  EdmLamp_D_Dsply/1 -> bus_creator/4  "EdmLamp_D_Dsply"
  EdmMsgTxt_D_Rq/1 -> bus_creator/5  "EdmMsgTxt_D_Rq"
  EdmPrev_Fe_Dsply/1 -> bus_creator/6  "EdmPrev_Fe_Dsply"
  EdmSailMdeOn_B_Stat/1 -> bus_creator/7  "EdmSailMdeOn_B_Stat"
  EdmVeh_V_Dsply/1 -> bus_creator/8  "EdmVeh_V_Dsply"

== system test_mdl1/VehicleCAN/ECM_Diesel/EngBrakeData ==
  AccEngStat_D_Actl : Constant  Value=0
  AccStopMde_D_Rq : Constant  Value=0
  BPedDrvAppl_D_QF : Constant  Value=0
  BpedDrvAppl_D_Actl : Constant  Value=0
  CcMde_D_Actl : Constant  Value=0
  CcOvrrdActv_B_Actl : Constant  Value=0
  CcStat_D_Actl : Constant  Value=0
  CmbbDeny_B_ActlPrpl : Constant  Value=0
  CmbbEngTqMn_B_Actl : Constant  Value=0
  EngAout_N_MnAllw : Constant  Value=0
  PrplTqMnSat_B_Actl : Constant  Value=0
  Veh_V_DsplyCcSet : Constant  Value=0
  bus_creator : BusCreator  Inputs=12
  out_port : Outport
  wires:
  bus_creator/1 -> out_port/1  "test_mdl1"
  AccEngStat_D_Actl/1 -> bus_creator/1  "AccEngStat_D_Actl"
  AccStopMde_D_Rq/1 -> bus_creator/2  "AccStopMde_D_Rq"
  BPedDrvAppl_D_QF/1 -> bus_creator/3  "BPedDrvAppl_D_QF"
  BpedDrvAppl_D_Actl/1 -> bus_creator/4  "BpedDrvAppl_D_Actl"
  CcMde_D_Actl/1 -> bus_creator/5  "CcMde_D_Actl"
  CcOvrrdActv_B_Actl/1 -> bus_creator/6  "CcOvrrdActv_B_Actl"
  CcStat_D_Actl/1 -> bus_creator/7  "CcStat_D_Actl"
  CmbbDeny_B_ActlPrpl/1 -> bus_creator/8  "CmbbDeny_B_ActlPrpl"
  CmbbEngTqMn_B_Actl/1 -> bus_creator/9  "CmbbEngTqMn_B_Actl"
  EngAout_N_MnAllw/1 -> bus_creator/10  "EngAout_N_MnAllw"
  PrplTqMnSat_B_Actl/1 -> bus_creator/11  "PrplTqMnSat_B_Actl"
  Veh_V_DsplyCcSet/1 -> bus_creator/12  "Veh_V_DsplyCcSet"

== system test_mdl1/VehicleCAN/ECM_Diesel/EngVehicleSpThrottle ==
  ApedPosPcActl_D_Qf : Constant  Value=0
  ApedPosPcActl_No_Cnt : Constant  Value=0
  ApedPosPcActl_No_Cs : Constant  Value=0
  ApedPos_PcRate_ActlArb : Constant  Value=0
  ApedPos_Pc_ActlArb : Constant  Value=0
  EngAout3_N_Actl : Constant  Value=0
  EngAoutNActl_D_QF : Constant  Value=0
  EngAout_N_Actl : Constant  Value=0
  bus_creator : BusCreator  Inputs=8
  out_port : Outport
  wires:
  bus_creator/1 -> out_port/1  "test_mdl1"
  ApedPosPcActl_D_Qf/1 -> bus_creator/1  "ApedPosPcActl_D_Qf"
  ApedPosPcActl_No_Cnt/1 -> bus_creator/2  "ApedPosPcActl_No_Cnt"
  ApedPosPcActl_No_Cs/1 -> bus_creator/3  "ApedPosPcActl_No_Cs"
  ApedPos_PcRate_ActlArb/1 -> bus_creator/4  "ApedPos_PcRate_ActlArb"
  ApedPos_Pc_ActlArb/1 -> bus_creator/5  "ApedPos_Pc_ActlArb"
  EngAout3_N_Actl/1 -> bus_creator/6  "EngAout3_N_Actl"
  EngAoutNActl_D_QF/1 -> bus_creator/7  "EngAoutNActl_D_QF"
  EngAout_N_Actl/1 -> bus_creator/8  "EngAout_N_Actl"

== system test_mdl1/VehicleCAN/ECM_Diesel/EngVehicleSpThrottle2 ==
  GearRvrse_D_Actl : Constant  Value=0
  StrtrMtrCtlMsgTxt_D2_Rq : Constant  Value=0
  StrtrMtrCtlMsgTxt_D_Rq : Constant  Value=0
  StrtrMtrDlyStrt_B_Stat : Constant  Value=0
  VehVActlEng_D_Qf : Constant  Value=0
  VehVActlEng_No_Cnt : Constant  Value=0
  VehVActlEng_No_Cs : Constant  Value=0
  VehVTrlrAid_B_Avail : Constant  Value=0
  Veh_V_ActlEng : Constant  Value=0
  Veh_V_RqCcSet : Constant  Value=0
  bus_creator : BusCreator  Inputs=10
  out_port : Outport
  wires:
  bus_creator/1 -> out_port/1  "test_mdl1"
  GearRvrse_D_Actl/1 -> bus_creator/1  "GearRvrse_D_Actl"
  StrtrMtrCtlMsgTxt_D2_Rq/1 -> bus_creator/2  "StrtrMtrCtlMsgTxt_D2_Rq"
  StrtrMtrCtlMsgTxt_D_Rq/1 -> bus_creator/3  "StrtrMtrCtlMsgTxt_D_Rq"
  StrtrMtrDlyStrt_B_Stat/1 -> bus_creator/4  "StrtrMtrDlyStrt_B_Stat"
  VehVActlEng_D_Qf/1 -> bus_creator/5  "VehVActlEng_D_Qf"
  VehVActlEng_No_Cnt/1 -> bus_creator/6  "VehVActlEng_No_Cnt"
  VehVActlEng_No_Cs/1 -> bus_creator/7  "VehVActlEng_No_Cs"
  VehVTrlrAid_B_Avail/1 -> bus_creator/8  "VehVTrlrAid_B_Avail"
  Veh_V_ActlEng/1 -> bus_creator/9  "Veh_V_ActlEng"
  Veh_V_RqCcSet/1 -> bus_creator/10  "Veh_V_RqCcSet"

== system test_mdl1/VehicleCAN/ECM_Diesel/EngineClimateData ==
  AirAmbTe_D_Qf : Constant  Value=0
  AirAmb_P_Actl : Constant  Value=0
  AirAmb_Te_Actl : Constant  Value=0
  AirAmb_Te_ActlFilt : Constant  Value=0
  AslChime_B_Rq : Constant  Value=0
  AslIconDsply_D_Rq : Constant  Value=0
  DynoMde_B_Cmd : Constant  Value=0
  EcssLamp_D_RqDsply : Constant  Value=0
  EngAout_Aa_Actl : Constant  Value=0
  GasPrtc_D_RqDsply : Constant  Value=0
  HvacHtrCore2_Te_Actl : Constant  Value=0
  bus_creator : BusCreator  Inputs=11
  out_port : Outport
  wires:
  bus_creator/1 -> out_port/1  "test_mdl1"
  AirAmbTe_D_Qf/1 -> bus_creator/1  "AirAmbTe_D_Qf"
  AirAmb_P_Actl/1 -> bus_creator/2  "AirAmb_P_Actl"
  AirAmb_Te_Actl/1 -> bus_creator/3  "AirAmb_Te_Actl"
  AirAmb_Te_ActlFilt/1 -> bus_creator/4  "AirAmb_Te_ActlFilt"
  AslChime_B_Rq/1 -> bus_creator/5  "AslChime_B_Rq"
  AslIconDsply_D_Rq/1 -> bus_creator/6  "AslIconDsply_D_Rq"
  DynoMde_B_Cmd/1 -> bus_creator/7  "DynoMde_B_Cmd"
  EcssLamp_D_RqDsply/1 -> bus_creator/8  "EcssLamp_D_RqDsply"
  EngAout_Aa_Actl/1 -> bus_creator/9  "EngAout_Aa_Actl"
  GasPrtc_D_RqDsply/1 -> bus_creator/10  "GasPrtc_D_RqDsply"
  HvacHtrCore2_Te_Actl/1 -> bus_creator/11  "HvacHtrCore2_Te_Actl"

== system test_mdl1/VehicleCAN/ECM_Diesel/EngineData_10 ==
  AccFllwMdeActv_B_Actl : Constant  Value=0
  AutoRgenTxt_B_RqDsply : Constant  Value=0
  DieslMsgTxt_D_Rq : Constant  Value=0
  EngPtoMde_D_Actl : Constant  Value=0
  ManRgenSoot_Pc_RqDsply : Constant  Value=0
  ManRgenTxt_D_RqDsply : Constant  Value=0
  bus_creator : BusCreator  Inputs=6
  out_port : Outport
  wires:
  bus_creator/1 -> out_port/1  "test_mdl1"
  AccFllwMdeActv_B_Actl/1 -> bus_creator/1  "AccFllwMdeActv_B_Actl"
  AutoRgenTxt_B_RqDsply/1 -> bus_creator/2  "AutoRgenTxt_B_RqDsply"
  DieslMsgTxt_D_Rq/1 -> bus_creator/3  "DieslMsgTxt_D_Rq"
  EngPtoMde_D_Actl/1 -> bus_creator/4  "EngPtoMde_D_Actl"
  ManRgenSoot_Pc_RqDsply/1 -> bus_creator/5  "ManRgenSoot_Pc_RqDsply"
  ManRgenTxt_D_RqDsply/1 -> bus_creator/6  "ManRgenTxt_D_RqDsply"

== system test_mdl1/VehicleCAN/ECM_Diesel/EngineData_11 ==
  DieslPrtc2_D_RqDsply : Constant  Value=0
  DieslPrtcRgen_D_Actl : Constant  Value=0
  EngExhOvrTe_B_RqDsply : Constant  Value=0
  EngTeColdPrtct_D_Stats : Constant  Value=0
  bus_creator : BusCreator  Inputs=4
  out_port : Outport
  wires:
  bus_creator/1 -> out_port/1  "test_mdl1"
  DieslPrtc2_D_RqDsply/1 -> bus_creator/1  "DieslPrtc2_D_RqDsply"
  DieslPrtcRgen_D_Actl/1 -> bus_creator/2  "DieslPrtcRgen_D_Actl"
  EngExhOvrTe_B_RqDsply/1 -> bus_creator/3  "EngExhOvrTe_B_RqDsply"
  EngTeColdPrtct_D_Stats/1 -> bus_creator/4  "EngTeColdPrtct_D_Stats"

== system test_mdl1/VehicleCAN/ECM_Diesel/EngineData_16 ==
  EngAout_N_MxAllw : Constant  Value=0
  EngExhBrkAutoLamp_B_Rq : Constant  Value=0
  EngExhBrkMde_D_Actl : Constant  Value=0
  EngExhBrkOnLamp_B_Rq : Constant  Value=0
  EngOilLvlWarn_D_Rq1 : Constant  Value=0
  bus_creator : BusCreator  Inputs=5
  out_port : Outport
  wires:
  bus_creator/1 -> out_port/1  "test_mdl1"
  EngAout_N_MxAllw/1 -> bus_creator/1  "EngAout_N_MxAllw"
  EngExhBrkAutoLamp_B_Rq/1 -> bus_creator/2  "EngExhBrkAutoLamp_B_Rq"
  EngExhBrkMde_D_Actl/1 -> bus_creator/3  "EngExhBrkMde_D_Actl"
  EngExhBrkOnLamp_B_Rq/1 -> bus_creator/4  "EngExhBrkOnLamp_B_Rq"
  EngOilLvlWarn_D_Rq1/1 -> bus_creator/5  "EngOilLvlWarn_D_Rq1"

== system test_mdl1/VehicleCAN/ECM_Diesel/EngineData_17 ==
  DistToNextOilChange : Constant  Value=0
  EngOilLife_T_Actl : Constant  Value=0
  EngOilSrvcMsgTxt_D_Rq : Constant  Value=0
  GlowIndication : Constant  Value=0
  RunDryPrevent_B_Stat : Constant  Value=0
  WaterInFuel : Constant  Value=0
  bus_creator : BusCreator  Inputs=6
  out_port : Outport
  wires:
  bus_creator/1 -> out_port/1  "test_mdl1"
  DistToNextOilChange/1 -> bus_creator/1  "DistToNextOilChange"
  EngOilLife_T_Actl/1 -> bus_creator/2  "EngOilLife_T_Actl"
  EngOilSrvcMsgTxt_D_Rq/1 -> bus_creator/3  "EngOilSrvcMsgTxt_D_Rq"
  GlowIndication/1 -> bus_creator/4  "GlowIndication"
  RunDryPrevent_B_Stat/1 -> bus_creator/5  "RunDryPrevent_B_Stat"
  WaterInFuel/1 -> bus_creator/6  "WaterInFuel"

== system test_mdl1/VehicleCAN/ECM_Diesel/EngineData_6 ==
  EngClntTe_D_Qf : Constant  Value=0
  EngClnt_Te_Actl : Constant  Value=0
  EngGoutLss_Tq_Est : Constant  Value=0
  EngOil_Te_Actl : Constant  Value=0
  EngOvrhtMitgActv_D_Ind : Constant  Value=0
  bus_creator : BusCreator  Inputs=5
  out_port : Outport
  wires:
  bus_creator/1 -> out_port/1  "test_mdl1"
  EngClntTe_D_Qf/1 -> bus_creator/1  "EngClntTe_D_Qf"
  EngClnt_Te_Actl/1 -> bus_creator/2  "EngClnt_Te_Actl"
  EngGoutLss_Tq_Est/1 -> bus_creator/3  "EngGoutLss_Tq_Est"
  EngOil_Te_Actl/1 -> bus_creator/4  "EngOil_Te_Actl"
  EngOvrhtMitgActv_D_Ind/1 -> bus_creator/5  "EngOvrhtMitgActv_D_Ind"

== system test_mdl1/VehicleCAN/ECM_Diesel/EngineData_7 ==
  AirCondClutch_B_Stats : Constant  Value=0
  AirCondRec_B_Rq : Constant  Value=0
  EngOilLife_Pc_Actl : Constant  Value=0
  EngSrvcRqd_B_Rq : Constant  Value=0
  FuelFillInlet_B_Dsply : Constant  Value=0
  FuelFilterLamp_B_Dsply : Constant  Value=0
  FuelFlw_Vl_Dsply : Constant  Value=0
  HvacAirFullOut_B_Rq : Constant  Value=0
  OdoCount : Constant  Value=0
  bus_creator : BusCreator  Inputs=9
  out_port : Outport
  wires:
  bus_creator/1 -> out_port/1  "test_mdl1"
  AirCondClutch_B_Stats/1 -> bus_creator/1  "AirCondClutch_B_Stats"
  AirCondRec_B_Rq/1 -> bus_creator/2  "AirCondRec_B_Rq"
  EngOilLife_Pc_Actl/1 -> bus_creator/3  "EngOilLife_Pc_Actl"
  EngSrvcRqd_B_Rq/1 -> bus_creator/4  "EngSrvcRqd_B_Rq"
  FuelFillInlet_B_Dsply/1 -> bus_creator/5  "FuelFillInlet_B_Dsply"
  FuelFilterLamp_B_Dsply/1 -> bus_creator/6  "FuelFilterLamp_B_Dsply"
  FuelFlw_Vl_Dsply/1 -> bus_creator/7  "FuelFlw_Vl_Dsply"
  HvacAirFullOut_B_Rq/1 -> bus_creator/8  "HvacAirFullOut_B_Rq"
  OdoCount/1 -> bus_creator/9  "OdoCount"

== system test_mdl1/VehicleCAN/ECM_Diesel/Engine_Clutch_Data ==
  CluPdlPosPcMeas_D_Qf : Constant  Value=0
  CluPdlPos_Pc_Meas : Constant  Value=0
  CluPdl_PcRate_Actl : Constant  Value=0
  EngAoutIdl_N_Ntrl : Constant  Value=0
  EngAout_N_Dsply : Constant  Value=0
  bus_creator : BusCreator  Inputs=5
  out_port : Outport
  wires:
  bus_creator/1 -> out_port/1  "test_mdl1"
  CluPdlPosPcMeas_D_Qf/1 -> bus_creator/1  "CluPdlPosPcMeas_D_Qf"
  CluPdlPos_Pc_Meas/1 -> bus_creator/2  "CluPdlPos_Pc_Meas"
  CluPdl_PcRate_Actl/1 -> bus_creator/3  "CluPdl_PcRate_Actl"
  EngAoutIdl_N_Ntrl/1 -> bus_creator/4  "EngAoutIdl_N_Ntrl"
  EngAout_N_Dsply/1 -> bus_creator/5  "EngAout_N_Dsply"

== system test_mdl1/VehicleCAN/ECM_Diesel/Engine_Data_18 ==
  EngAirFiltMsgTxt_D_Rq : Constant  Value=0
  UreaMnAdd_L2_Actl : Constant  Value=0
  UreaMxAdd_L2_Actl : Constant  Value=0
  VehUreaRnge3_L_DsplyMx : Constant  Value=0
  WaterInFuel_B_Falt : Constant  Value=0
  bus_creator : BusCreator  Inputs=5
  out_port : Outport
  wires:
  bus_creator/1 -> out_port/1  "test_mdl1"
  EngAirFiltMsgTxt_D_Rq/1 -> bus_creator/1  "EngAirFiltMsgTxt_D_Rq"
  UreaMnAdd_L2_Actl/1 -> bus_creator/2  "UreaMnAdd_L2_Actl"
  UreaMxAdd_L2_Actl/1 -> bus_creator/3  "UreaMxAdd_L2_Actl"
  VehUreaRnge3_L_DsplyMx/1 -> bus_creator/4  "VehUreaRnge3_L_DsplyMx"
  WaterInFuel_B_Falt/1 -> bus_creator/5  "WaterInFuel_B_Falt"

== system test_mdl1/VehicleCAN/ECM_Diesel/Global_PATS_TargetInfo ==
  bus_creator : BusCreator  Inputs=3
  immoTarget1Cmd : Constant  Value=0
  immoTarget1Data : Constant  Value=0
  immoTarget1Status : Constant  Value=0
  out_port : Outport
  wires:
  bus_creator/1 -> out_port/1  "test_mdl1"
  immoTarget1Cmd/1 -> bus_creator/1  "immoTarget1Cmd"
  immoTarget1Data/1 -> bus_creator/2  "immoTarget1Data"
  immoTarget1Status/1 -> bus_creator/3  "immoTarget1Status"

== system test_mdl1/VehicleCAN/ECM_Diesel/Low_Voltage_Power_Data_FD1 ==
  PwSrcULoComm_B_Falt : Constant  Value=0
  PwSrcULoDcnnt_B_Stat : Constant  Value=0
  PwSrcULoFalt_D_Stat : Constant  Value=0
  PwSrcULoOvrTe_B_Actl : Constant  Value=0
  PwSrcULo_I_Actl : Constant  Value=0
  PwSrcULo_I_Mx : Constant  Value=0
  PwSrcULo_Pc_Mx : Constant  Value=0
  ULoRgenTestMde_B_Stat : Constant  Value=0
  bus_creator : BusCreator  Inputs=8
  out_port : Outport
  wires:
  bus_creator/1 -> out_port/1  "test_mdl1"
  PwSrcULoComm_B_Falt/1 -> bus_creator/1  "PwSrcULoComm_B_Falt"
  PwSrcULoDcnnt_B_Stat/1 -> bus_creator/2  "PwSrcULoDcnnt_B_Stat"
  PwSrcULoFalt_D_Stat/1 -> bus_creator/3  "PwSrcULoFalt_D_Stat"
  PwSrcULoOvrTe_B_Actl/1 -> bus_creator/4  "PwSrcULoOvrTe_B_Actl"
  PwSrcULo_I_Actl/1 -> bus_creator/5  "PwSrcULo_I_Actl"
  PwSrcULo_I_Mx/1 -> bus_creator/6  "PwSrcULo_I_Mx"
  PwSrcULo_Pc_Mx/1 -> bus_creator/7  "PwSrcULo_Pc_Mx"
  ULoRgenTestMde_B_Stat/1 -> bus_creator/8  "ULoRgenTestMde_B_Stat"

== system test_mdl1/VehicleCAN/ECM_Diesel/OTAPhysPCMtoGWM_ECG ==
  OTAPhysPCMtoGWM_ECG : Constant  Value=0
  bus_creator : BusCreator  Inputs=1
  out_port : Outport
  wires:
  bus_creator/1 -> out_port/1  "test_mdl1"
  OTAPhysPCMtoGWM_ECG/1 -> bus_creator/1  "OTAPhysPCMtoGWM_ECG"

== system test_mdl1/VehicleCAN/ECM_Diesel/PARSEDPhysPCMtoGWM_ECG ==
  PARSEDPhysPCMtoGWM_ECG : Constant  Value=0
  bus_creator : BusCreator  Inputs=1
  out_port : Outport
  wires:
  bus_creator/1 -> out_port/1  "test_mdl1"
  PARSEDPhysPCMtoGWM_ECG/1 -> bus_creator/1  "PARSEDPhysPCMtoGWM_ECG"

== system test_mdl1/VehicleCAN/ECM_Diesel/PARSEDPushPCMtoGWM_ECG ==
  PARSEDPushPCMtoGWM_ECG : Constant  Value=0
  bus_creator : BusCreator  Inputs=1
  out_port : Outport
  wires:
  bus_creator/1 -> out_port/1  "test_mdl1"
  PARSEDPushPCMtoGWM_ECG/1 -> bus_creator/1  "PARSEDPushPCMtoGWM_ECG"

== system test_mdl1/VehicleCAN/ECM_Diesel/PCM_AutoSar_NetworkMgmt ==
  PCM_AutoSarNMControl : Constant  Value=0
  PCM_AutoSarNMNodeId : Constant  Value=0
  PCM_AutoSarNMReserved{1..4} (4 alike) : Constant  Value=0
  PCM_GWNMProxy : Constant  Value=0
  PCM_GWOnBoardTester : Constant  Value=0
  bus_creator : BusCreator  Inputs=8
  out_port : Outport
  wires:
  bus_creator/1 -> out_port/1  "test_mdl1"
  PCM_AutoSarNMControl/1 -> bus_creator/1  "PCM_AutoSarNMControl"
  PCM_AutoSarNMNodeId/1 -> bus_creator/2  "PCM_AutoSarNMNodeId"
  PCM_AutoSarNMReserved1/1 -> bus_creator/3  "PCM_AutoSarNMReserved1"
  PCM_AutoSarNMReserved2/1 -> bus_creator/4  "PCM_AutoSarNMReserved2"
  PCM_AutoSarNMReserved3/1 -> bus_creator/5  "PCM_AutoSarNMReserved3"
  PCM_AutoSarNMReserved4/1 -> bus_creator/6  "PCM_AutoSarNMReserved4"
  PCM_GWNMProxy/1 -> bus_creator/7  "PCM_GWNMProxy"
  PCM_GWOnBoardTester/1 -> bus_creator/8  "PCM_GWOnBoardTester"

== system test_mdl1/VehicleCAN/ECM_Diesel/PCM_Rapid_Data_Response_1 ==
  UUDTPCMResponse1 : Constant  Value=0
  bus_creator : BusCreator  Inputs=1
  out_port : Outport
  wires:
  bus_creator/1 -> out_port/1  "test_mdl1"
  UUDTPCMResponse1/1 -> bus_creator/1  "UUDTPCMResponse1"

== system test_mdl1/VehicleCAN/ECM_Diesel/PCM_Rapid_Data_Response_2 ==
  UUDTPCMResponse2 : Constant  Value=0
  bus_creator : BusCreator  Inputs=1
  out_port : Outport
  wires:
  bus_creator/1 -> out_port/1  "test_mdl1"
  UUDTPCMResponse2/1 -> bus_creator/1  "UUDTPCMResponse2"

== system test_mdl1/VehicleCAN/ECM_Diesel/PowertrainData_1 ==
  AirCondFluidHi_P_Actl : Constant  Value=0
  CoolantFanStepAct : Constant  Value=0
  ECMMILRequest : Constant  Value=0
  EngIdlShutDown_D_Stat : Constant  Value=0
  EngIdlShutDwnTxt_D_Rq : Constant  Value=0
  FUEL_ALCOHOL_PERCNT : Constant  Value=0
  FohEng_D_Rq : Constant  Value=0
  OilPressureWarning : Constant  Value=0
  TrnTotLss_Tq_Est : Constant  Value=0
  TrnTotTq_Rt_Est : Constant  Value=0
  VehVLimActv_B_Actl : Constant  Value=0
  VehVLimStat_D_Actl : Constant  Value=0
  bus_creator : BusCreator  Inputs=12
  out_port : Outport
  wires:
  bus_creator/1 -> out_port/1  "test_mdl1"
  AirCondFluidHi_P_Actl/1 -> bus_creator/1  "AirCondFluidHi_P_Actl"
  CoolantFanStepAct/1 -> bus_creator/2  "CoolantFanStepAct"
  ECMMILRequest/1 -> bus_creator/3  "ECMMILRequest"
  EngIdlShutDown_D_Stat/1 -> bus_creator/4  "EngIdlShutDown_D_Stat"
  EngIdlShutDwnTxt_D_Rq/1 -> bus_creator/5  "EngIdlShutDwnTxt_D_Rq"
  FUEL_ALCOHOL_PERCNT/1 -> bus_creator/6  "FUEL_ALCOHOL_PERCNT"
  FohEng_D_Rq/1 -> bus_creator/7  "FohEng_D_Rq"
  OilPressureWarning/1 -> bus_creator/8  "OilPressureWarning"
  TrnTotLss_Tq_Est/1 -> bus_creator/9  "TrnTotLss_Tq_Est"
  TrnTotTq_Rt_Est/1 -> bus_creator/10  "TrnTotTq_Rt_Est"
  VehVLimActv_B_Actl/1 -> bus_creator/11  "VehVLimActv_B_Actl"
  VehVLimStat_D_Actl/1 -> bus_creator/12  "VehVLimStat_D_Actl"

== system test_mdl1/VehicleCAN/ECM_Diesel/PowertrainData_11 ==
  GearNtrl_D_Stat : Constant  Value=0
  GearNtrl_No_Cnt : Constant  Value=0
  GearNtrl_No_Cs : Constant  Value=0
  bus_creator : BusCreator  Inputs=3
  out_port : Outport
  wires:
  bus_creator/1 -> out_port/1  "test_mdl1"
  GearNtrl_D_Stat/1 -> bus_creator/1  "GearNtrl_D_Stat"
  GearNtrl_No_Cnt/1 -> bus_creator/2  "GearNtrl_No_Cnt"
  GearNtrl_No_Cs/1 -> bus_creator/3  "GearNtrl_No_Cs"

== system test_mdl1/VehicleCAN/ECM_Diesel/PowertrainData_12 ==
  PtIgnSwtch_D_Stat : Constant  Value=0
  PtIgnSwtch_No_Cnt : Constant  Value=0
  PtIgnSwtch_No_Cs : Constant  Value=0
  bus_creator : BusCreator  Inputs=3
  out_port : Outport
  wires:
  bus_creator/1 -> out_port/1  "test_mdl1"
  PtIgnSwtch_D_Stat/1 -> bus_creator/1  "PtIgnSwtch_D_Stat"
  PtIgnSwtch_No_Cnt/1 -> bus_creator/2  "PtIgnSwtch_No_Cnt"
  PtIgnSwtch_No_Cs/1 -> bus_creator/3  "PtIgnSwtch_No_Cs"

== system test_mdl1/VehicleCAN/ECM_Diesel/PowertrainData_2 ==
  ApedPos_Pc_ActlDiag : Constant  Value=0
  EngAirIn_Te_Actl : Constant  Value=0
  EngClnt_Te_ActlDiag : Constant  Value=0
  EngLoad_Pc_CalcDiag : Constant  Value=0
  EngMsgTxt_D_Rq : Constant  Value=0
  GrllShtrPos_B_Falt : Constant  Value=0
  GrllShtrPos_D_Cmd : Constant  Value=0
  IsaOffst_D_Stat : Constant  Value=0
  ObdWarmUp_B_Complt : Constant  Value=0
  SlMde_D_RqDsply : Constant  Value=0
  SlMde_D_Stat : Constant  Value=0
  bus_creator : BusCreator  Inputs=11
  out_port : Outport
  wires:
  bus_creator/1 -> out_port/1  "test_mdl1"
  ApedPos_Pc_ActlDiag/1 -> bus_creator/1  "ApedPos_Pc_ActlDiag"
  EngAirIn_Te_Actl/1 -> bus_creator/2  "EngAirIn_Te_Actl"
  EngClnt_Te_ActlDiag/1 -> bus_creator/3  "EngClnt_Te_ActlDiag"
  EngLoad_Pc_CalcDiag/1 -> bus_creator/4  "EngLoad_Pc_CalcDiag"
  EngMsgTxt_D_Rq/1 -> bus_creator/5  "EngMsgTxt_D_Rq"
  GrllShtrPos_B_Falt/1 -> bus_creator/6  "GrllShtrPos_B_Falt"
  GrllShtrPos_D_Cmd/1 -> bus_creator/7  "GrllShtrPos_D_Cmd"
  IsaOffst_D_Stat/1 -> bus_creator/8  "IsaOffst_D_Stat"
  ObdWarmUp_B_Complt/1 -> bus_creator/9  "ObdWarmUp_B_Complt"
  SlMde_D_RqDsply/1 -> bus_creator/10  "SlMde_D_RqDsply"
  SlMde_D_Stat/1 -> bus_creator/11  "SlMde_D_Stat"

== system test_mdl1/VehicleCAN/ECM_Diesel/PowertrainData_3 ==
  BattULoChrg_U_Cmd : Constant  Value=0
  ElLoadCtl_D_Rq : Constant  Value=0
  EngMnfld_P_Actl : Constant  Value=0
  FuelPumpPwr_B_Rq : Constant  Value=0
  bus_creator : BusCreator  Inputs=4
  out_port : Outport
  wires:
  bus_creator/1 -> out_port/1  "test_mdl1"
  BattULoChrg_U_Cmd/1 -> bus_creator/1  "BattULoChrg_U_Cmd"
  ElLoadCtl_D_Rq/1 -> bus_creator/2  "ElLoadCtl_D_Rq"
  EngMnfld_P_Actl/1 -> bus_creator/3  "EngMnfld_P_Actl"
  FuelPumpPwr_B_Rq/1 -> bus_creator/4  "FuelPumpPwr_B_Rq"

== system test_mdl1/VehicleCAN/ECM_Diesel/PowertrainData_6 ==
  BrkTot_Tq_RqFapLc : Constant  Value=0
  FapLc_B_Err : Constant  Value=0
  TrnAin_Pc_RqDrv : Constant  Value=0
  bus_creator : BusCreator  Inputs=3
  out_port : Outport
  wires:
  bus_creator/1 -> out_port/1  "test_mdl1"
  BrkTot_Tq_RqFapLc/1 -> bus_creator/1  "BrkTot_Tq_RqFapLc"
  FapLc_B_Err/1 -> bus_creator/2  "FapLc_B_Err"
  TrnAin_Pc_RqDrv/1 -> bus_creator/3  "TrnAin_Pc_RqDrv"

== system test_mdl1/VehicleCAN/ECM_Diesel/PowertrainData_7 ==
  EcoCochA_Pc_Dsply : Constant  Value=0
  EcoCochCrus_Pc_Dsply : Constant  Value=0
  EcoCochDecel_Pc_Dsply : Constant  Value=0
  EcoCochIdlFuel_Pc_Dsply : Constant  Value=0
  EcoCochInstNeg_B_Dsply : Constant  Value=0
  EcoCochInst_Pc_Dsply : Constant  Value=0
  EcoCochShif_Pc_Dsply : Constant  Value=0
  bus_creator : BusCreator  Inputs=7
  out_port : Outport
  wires:
  bus_creator/1 -> out_port/1  "test_mdl1"
  EcoCochA_Pc_Dsply/1 -> bus_creator/1  "EcoCochA_Pc_Dsply"
  EcoCochCrus_Pc_Dsply/1 -> bus_creator/2  "EcoCochCrus_Pc_Dsply"
  EcoCochDecel_Pc_Dsply/1 -> bus_creator/3  "EcoCochDecel_Pc_Dsply"
  EcoCochIdlFuel_Pc_Dsply/1 -> bus_creator/4  "EcoCochIdlFuel_Pc_Dsply"
  EcoCochInstNeg_B_Dsply/1 -> bus_creator/5  "EcoCochInstNeg_B_Dsply"
  EcoCochInst_Pc_Dsply/1 -> bus_creator/6  "EcoCochInst_Pc_Dsply"
  EcoCochShif_Pc_Dsply/1 -> bus_creator/7  "EcoCochShif_Pc_Dsply"

== system test_mdl1/VehicleCAN/ECM_Diesel/PowertrainData_9 ==
  AutoTowActv_B_Stat : Constant  Value=0
  AutoTowAllw_D_StatMnu : Constant  Value=0
  EngExhMdeQuiet_D2_Stat : Constant  Value=0
  GrossTrainWeight_M_Est : Constant  Value=0
  HvacCmprLim_D_Stat : Constant  Value=0
  TrailCtlPt_B_Falt : Constant  Value=0
  Veh_V_DsplyTrailCtlSet : Constant  Value=0
  WakeAlarm1_B_Typ : Constant  Value=0
  WakeAlarm1_T_Rq : Constant  Value=0
  bus_creator : BusCreator  Inputs=9
  out_port : Outport
  wires:
  bus_creator/1 -> out_port/1  "test_mdl1"
  AutoTowActv_B_Stat/1 -> bus_creator/1  "AutoTowActv_B_Stat"
  AutoTowAllw_D_StatMnu/1 -> bus_creator/2  "AutoTowAllw_D_StatMnu"
  EngExhMdeQuiet_D2_Stat/1 -> bus_creator/3  "EngExhMdeQuiet_D2_Stat"
  GrossTrainWeight_M_Est/1 -> bus_creator/4  "GrossTrainWeight_M_Est"
  HvacCmprLim_D_Stat/1 -> bus_creator/5  "HvacCmprLim_D_Stat"
  TrailCtlPt_B_Falt/1 -> bus_creator/6  "TrailCtlPt_B_Falt"
  Veh_V_DsplyTrailCtlSet/1 -> bus_creator/7  "Veh_V_DsplyTrailCtlSet"
  WakeAlarm1_B_Typ/1 -> bus_creator/8  "WakeAlarm1_B_Typ"
  WakeAlarm1_T_Rq/1 -> bus_creator/9  "WakeAlarm1_T_Rq"

== system test_mdl1/VehicleCAN/ECM_Diesel/Powertrain_Data_4 ==
  BpedDrvMsgTxt_B_Dsply : Constant  Value=0
  FuelLvlWarn_D_ActlEng : Constant  Value=0
  FuelLvl_Pc_DsplyEng : Constant  Value=0
  FuelRange_L_DsplyEng : Constant  Value=0
  RearDiffOilTeWarn_B_Rq : Constant  Value=0
  RearDiffOil_Te_Actl : Constant  Value=0
  SelDrvMdePt_D_Stat : Constant  Value=0
  bus_creator : BusCreator  Inputs=7
  out_port : Outport
  wires:
  bus_creator/1 -> out_port/1  "test_mdl1"
  BpedDrvMsgTxt_B_Dsply/1 -> bus_creator/1  "BpedDrvMsgTxt_B_Dsply"
  FuelLvlWarn_D_ActlEng/1 -> bus_creator/2  "FuelLvlWarn_D_ActlEng"
  FuelLvl_Pc_DsplyEng/1 -> bus_creator/3  "FuelLvl_Pc_DsplyEng"
  FuelRange_L_DsplyEng/1 -> bus_creator/4  "FuelRange_L_DsplyEng"
  RearDiffOilTeWarn_B_Rq/1 -> bus_creator/5  "RearDiffOilTeWarn_B_Rq"
  RearDiffOil_Te_Actl/1 -> bus_creator/6  "RearDiffOil_Te_Actl"
  SelDrvMdePt_D_Stat/1 -> bus_creator/7  "SelDrvMdePt_D_Stat"

== system test_mdl1/VehicleCAN/ECM_Diesel/Powertrain_Data_5 ==
  AdasLcObtclAbrt_B_Stat : Constant  Value=0
  AirDamPos_D_Stat : Constant  Value=0
  BattRgenLoChrg_D_RqEng : Constant  Value=0
  BattRgenLoDChrg_D_RqEng : Constant  Value=0
  FapLcActv_B_Stat : Constant  Value=0
  FapLcInhbt_B_Rq : Constant  Value=0
  FapLcMaxGrdAbrt_B_Stat : Constant  Value=0
  FapLcMaxGrdInhbt_B_Stat : Constant  Value=0
  FapLcObstcl_B_Stat : Constant  Value=0
  FapLcPrchgBrk_B_Rq : Constant  Value=0
  FapLcStopHold_B_Rq : Constant  Value=0
  bus_creator : BusCreator  Inputs=11
  out_port : Outport
  wires:
  bus_creator/1 -> out_port/1  "test_mdl1"
  AdasLcObtclAbrt_B_Stat/1 -> bus_creator/1  "AdasLcObtclAbrt_B_Stat"
  AirDamPos_D_Stat/1 -> bus_creator/2  "AirDamPos_D_Stat"
  BattRgenLoChrg_D_RqEng/1 -> bus_creator/3  "BattRgenLoChrg_D_RqEng"
  BattRgenLoDChrg_D_RqEng/1 -> bus_creator/4  "BattRgenLoDChrg_D_RqEng"
  FapLcActv_B_Stat/1 -> bus_creator/5  "FapLcActv_B_Stat"
  FapLcInhbt_B_Rq/1 -> bus_creator/6  "FapLcInhbt_B_Rq"
  FapLcMaxGrdAbrt_B_Stat/1 -> bus_creator/7  "FapLcMaxGrdAbrt_B_Stat"
  FapLcMaxGrdInhbt_B_Stat/1 -> bus_creator/8  "FapLcMaxGrdInhbt_B_Stat"
  FapLcObstcl_B_Stat/1 -> bus_creator/9  "FapLcObstcl_B_Stat"
  FapLcPrchgBrk_B_Rq/1 -> bus_creator/10  "FapLcPrchgBrk_B_Rq"
  FapLcStopHold_B_Rq/1 -> bus_creator/11  "FapLcStopHold_B_Rq"
